simulink model "AGC"  (R2022a)
settings: Solver=FixedStepAuto  StartTime=0.0  StopTime=8000/Fs  RelTol=1e-3
undefined symbols (not defined in the file): a, alpha, Fixeda, FixedR, Fs, magnitude, R, TimeAxis
libraries: sim_stud_lib_r2022a x13, dspswit3 x2
settings Model: Creator=RolePyps  LastModifiedBy=RolePups
settings DebuggingCC: ParameterPrecisionLossMsg=none

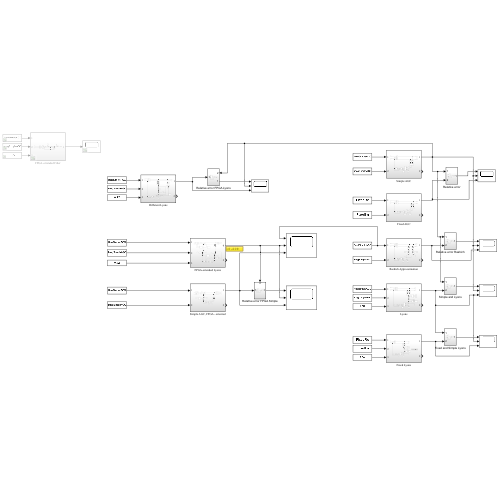
[thumbnail: Simulink's stored preview of the top-level diagram]
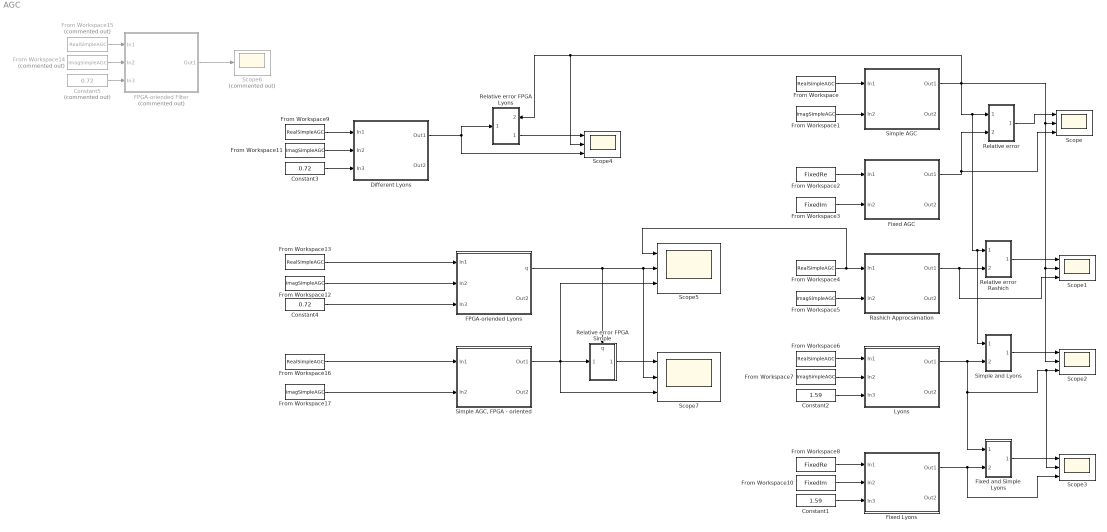
== system AGC ==
  Constant1 : Constant  Value=1.59  OutDataTypeStr=fixdt(0,13,11)  SampleTime=-1
  Constant2 : Constant  Value=1.59  SampleTime=1/Fs
  Constant3 : Constant  Value=0.72  SampleTime=1/Fs
  Constant4 : Constant  Value=0.72  SampleTime=TimeAxis(2)
  Constant5 : Constant  Commented=on  Value=0.72  SampleTime=1/Fs
  Different Lyons : Subsystem
  FPGA-oriended Filter : Subsystem  Commented=on
  FPGA-oriended Lyons : Subsystem
  Fixed AGC : Subsystem
  Fixed Lyons : Subsystem
  Fixed and Simple Lyons : Subsystem
  From Workspace{,4,6,9} (4 alike) : FromWorkspace  VariableName=RealSimpleAGC  OutDataTypeStr=double  SampleTime=1/Fs  Interpolate=off  OutputAfterFinalValue=Setting to zero
  From Workspace{1,5,7,11} (4 alike) : FromWorkspace  VariableName=ImagSimpleAGC  SampleTime=1/Fs  Interpolate=off  OutputAfterFinalValue=Setting to zero
  From Workspace10 : FromWorkspace  VariableName=FixedIm  OutDataTypeStr=fixdt(1,16,14)  SampleTime=1/Fs  Interpolate=off  OutputAfterFinalValue=Setting to zero
  From Workspace12 : FromWorkspace  VariableName=ImagSimpleAGC  SampleTime=TimeAxis(2)  Interpolate=off  OutputAfterFinalValue=Setting to zero
  From Workspace13 : FromWorkspace  VariableName=RealSimpleAGC  SampleTime=TimeAxis(2)  Interpolate=off  OutputAfterFinalValue=Setting to zero
  From Workspace14 : FromWorkspace  Commented=on  VariableName=ImagSimpleAGC  SampleTime=1/Fs  Interpolate=off  OutputAfterFinalValue=Setting to zero
  From Workspace15 : FromWorkspace  Commented=on  VariableName=RealSimpleAGC  OutDataTypeStr=double  SampleTime=1/Fs  Interpolate=off  OutputAfterFinalValue=Setting to zero
  From Workspace16 : FromWorkspace  VariableName=RealSimpleAGC  OutDataTypeStr=double  SampleTime=40/Fs  Interpolate=off  OutputAfterFinalValue=Setting to zero
  From Workspace17 : FromWorkspace  VariableName=ImagSimpleAGC  SampleTime=40/Fs  Interpolate=off  OutputAfterFinalValue=Setting to zero
  From Workspace2 : FromWorkspace  VariableName=FixedRe  OutDataTypeStr=fixdt(1,16,14)  SampleTime=1/Fs  Interpolate=off  OutputAfterFinalValue=Setting to zero
  From Workspace3 : FromWorkspace  VariableName=FixedIm  OutDataTypeStr=fixdt(1,16,14)  SampleTime=1/Fs  Interpolate=off  OutputAfterFinalValue=Setting to zero
  From Workspace8 : FromWorkspace  VariableName=FixedRe  OutDataTypeStr=fixdt(1,16,14)  SampleTime=1/Fs  Interpolate=off  OutputAfterFinalValue=Setting to zero
  Lyons : Subsystem
  Rashich Approcsimation : Subsystem
  Relative error : Subsystem
  Relative error FPGA Lyons : Subsystem
      settings: PortSchema="{\"entries\":[{\"content\":{\"sides\":[{\"content\":{\"connectorIds\":[\"In1\"]},\"type\":\"ConnectorPlacement.EquallySpacedRectSide\",\"uuid\":\"ab41bc29-8a88-48da-842a-7ea4b5d94515\"},{\"content\":{\"connectorIds\":[\"In2\",\"Out1\"],\"side\":\"RIGHT\"},\"type\":\"ConnectorPlacement.EquallySpacedRectSide\",\"uuid\":\"822f6f2f-923d-401a-b739-761bcd6fc88d\"},{\"content\":{\"connectorIds\":[],\"side\":\"TOP\"},\"type\":\"ConnectorPlacement.EquallySpacedRectSide\",\"uuid\":\"c3246772-222e-4e0d-9f9e-d4db37fa2bf2\"}]},\"type\":\"ConnectorPlacement.EquallySpacedConnector\",\"uuid\":\"7042a765-ada9-4885-ac85-35a265789643\"}],\"packageUris\":[\"http://schema.mathworks.com/mf0/Connector/R2020b\"],\"version\":\"1.0\"}"
  Relative error FPGA Simple : Subsystem
      settings: PortSchema="{\"entries\":[{\"content\":{\"sides\":[{\"content\":{\"connectorIds\":[\"In1\"]},\"type\":\"ConnectorPlacement.EquallySpacedRectSide\",\"uuid\":\"ab41bc29-8a88-48da-842a-7ea4b5d94515\"},{\"content\":{\"connectorIds\":[\"Out1\"],\"side\":\"RIGHT\"},\"type\":\"ConnectorPlacement.EquallySpacedRectSide\",\"uuid\":\"822f6f2f-923d-401a-b739-761bcd6fc88d\"},{\"content\":{\"connectorIds\":[\"In2\"],\"side\":\"TOP\"},\"type\":\"ConnectorPlacement.EquallySpacedRectSide\",\"uuid\":\"c3246772-222e-4e0d-9f9e-d4db37fa2bf2\"}]},\"type\":\"ConnectorPlacement.EquallySpacedConnector\",\"uuid\":\"7042a765-ada9-4885-ac85-35a265789643\"}],\"packageUris\":[\"http://schema.mathworks.com/mf0/Connector/R2020b\"],\"version\":\"1.0\"}"
  Relative error Rashich : Subsystem
  Scope{,1..5,7} (7 alike) : Scope  NumInputPorts=3
  Scope6 : Scope  Commented=on
  Simple AGC : Subsystem
  "Simple AGC, FPGA - oriented" : Subsystem
  Simple and Lyons : Subsystem
  wires:
  From Workspace/1 -> Simple AGC/1(In1)
  From Workspace1/1 -> Simple AGC/2(In2)
  Relative error/1(Out1) -> Scope/1
  From Workspace3/1 -> Fixed AGC/2(In2)
  From Workspace2/1 -> Fixed AGC/1(In1)
  Fixed AGC/1(Out1) -> Scope/3, Relative error/2(In3)
  From Workspace4/1 -> Scope5/1, Rashich Approcsimation/1(In1)
  From Workspace5/1 -> Rashich Approcsimation/2(In2)
  Rashich Approcsimation/1(Out1) -> Scope1/3, Relative error Rashich/2(In3)
  From Workspace6/1 -> Lyons/1(In1)
  From Workspace7/1 -> Lyons/2(In2)
  Lyons/1(Out1) -> Simple and Lyons/2(In3), Fixed and Simple Lyons/1(In1), Scope3/2, Scope2/3
  Simple and Lyons/1(Out1) -> Scope2/1
  Constant2/1 -> Lyons/3(In3)
  From Workspace8/1 -> Fixed Lyons/1(In1)
  Fixed Lyons/1(Out1) -> Fixed and Simple Lyons/2(In3), Scope3/3
  Constant1/1 -> Fixed Lyons/3(In3)
  From Workspace10/1 -> Fixed Lyons/2(In2)
  Fixed and Simple Lyons/1(Out1) -> Scope3/1
  Relative error Rashich/1(Out1) -> Scope1/1
  From Workspace11/1 -> Different Lyons/2(In2)
  Constant3/1 -> Different Lyons/3(In3)
  From Workspace9/1 -> Different Lyons/1(In1)
  Different Lyons/1(Out1) -> Scope4/3, Relative error FPGA Lyons/1(In3)
  Relative error FPGA Lyons/1(Out1) -> Scope4/1
  Constant4/1 -> FPGA-oriended Lyons/3(In3)
  From Workspace12/1 -> FPGA-oriended Lyons/2(In2)
  From Workspace15/1 -> FPGA-oriended Filter/1(In1)
  From Workspace14/1 -> FPGA-oriended Filter/2(In2)
  Constant5/1 -> FPGA-oriended Filter/3(In3)
  FPGA-oriended Filter/1(Out1) -> Scope6/1
  Simple AGC/1(Out1) -> Scope4/2, Relative error FPGA Lyons/2(In1), Scope2/2, Scope1/2, Scope/2, Simple and Lyons/1(In1), Relative error Rashich/1(In1), Relative error/1(In1)
  From Workspace13/1 -> FPGA-oriended Lyons/1(In1)
  FPGA-oriended Lyons/1(q) -> Relative error FPGA Simple/2(q), Scope7/2, Scope5/2
  From Workspace17/1 -> "Simple AGC, FPGA - oriented"/2(In2)
  From Workspace16/1 -> "Simple AGC, FPGA - oriented"/1(In1)
  "Simple AGC, FPGA - oriented"/1(Out1) -> Scope7/3, Relative error FPGA Simple/1(In3), Scope5/3
  Relative error FPGA Simple/1(Out1) -> Scope7/1

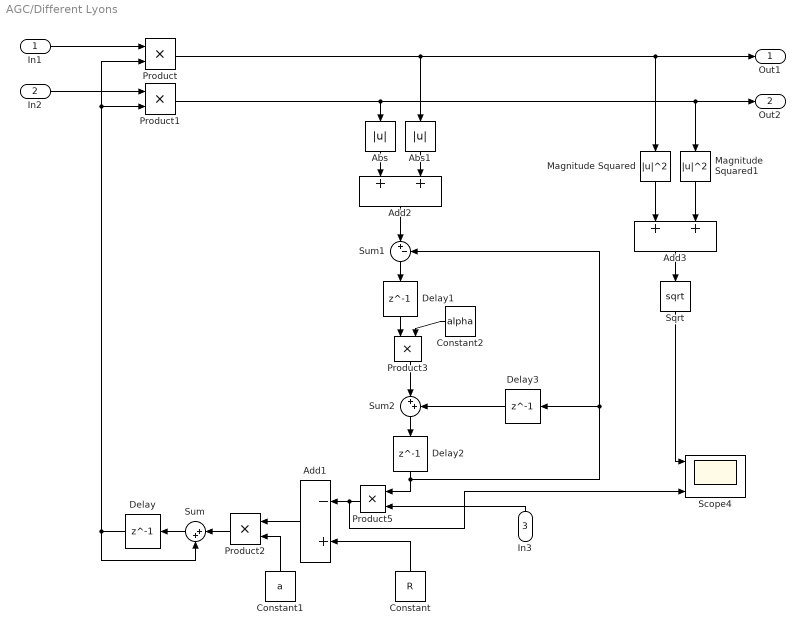
== system AGC/Different Lyons ==
  In1 : Inport
  In2 : Inport  Port=2
  In3 : Inport  Port=3  SampleTime=1/Fs
  Abs : Abs  SaturateOnIntegerOverflow=off
  Abs1 : Abs  SaturateOnIntegerOverflow=off
  Add1 : Sum  Inputs=-+  AccumDataTypeStr=double
  Add2 : Sum  AccumDataTypeStr=double
  Add3 : Sum  AccumDataTypeStr=double
  Constant : Constant  Value=R
  Constant1 : Constant  Value=a
  Constant2 : Constant  Value=alpha
  Delay{,1..3} (4 alike) : Delay  DelayLength=1  InitialCondition=0
  Magnitude Squared : Math  Operator=magnitude^2
  Magnitude Squared1 : Math  Operator=magnitude^2
  Product{,1..3,5} (5 alike) : Product  OutDataTypeStr=double
  Scope4 : Scope  NumInputPorts=3
  Sqrt : Sqrt
  Sum : Sum  Inputs=|++  AccumDataTypeStr=double
  Sum1 : Sum  Inputs=|+-  AccumDataTypeStr=double
  Sum2 : Sum  Inputs=|++  AccumDataTypeStr=double
  Out1 : Outport
  Out2 : Outport  Port=2
  wires:
  Delay/1 -> Sum/2, Product1/2, Product/2
  Product/1 -> Magnitude Squared/1, Out1/1, Abs1/1
  Add1/1 -> Product2/1
  Product1/1 -> Abs/1, Magnitude Squared1/1, Out2/1
  Constant/1 -> Add1/2
  In1/1 -> Product/1
  In2/1 -> Product1/1
  Sum/1 -> Delay/1
  Product2/1 -> Sum/1
  Constant1/1 -> Product2/2
  Abs1/1 -> Add2/2
  Abs/1 -> Add2/1
  In3/1 -> Product5/2
  Sum1/1 -> Delay1/1
  Product5/1 -> Scope4/3, Add1/1
  Add2/1 -> Sum1/1
  Delay1/1 -> Product3/1
  Constant2/1 -> Product3/2
  Product3/1 -> Sum2/1
  Sum2/1 -> Delay2/1
  Delay2/1 -> Delay3/1, Sum1/2, Product5/1
  Delay3/1 -> Sum2/2
  Magnitude Squared1/1 -> Add3/2
  Magnitude Squared/1 -> Add3/1
  Add3/1 -> Sqrt/1
  Sqrt/1 -> Scope4/1

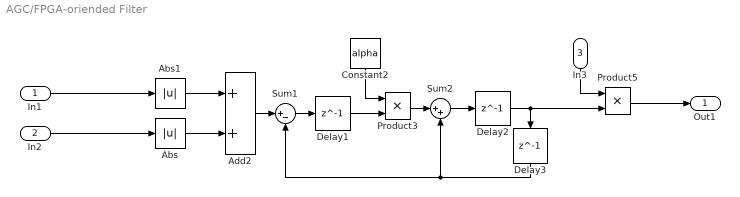
== system AGC/FPGA-oriended Filter ==
  In1 : Inport
  In2 : Inport  Port=2
  In3 : Inport  Port=3  SampleTime=1/Fs
  Abs : Abs  SaturateOnIntegerOverflow=off
  Abs1 : Abs  SaturateOnIntegerOverflow=off
  Add2 : Sum  AccumDataTypeStr=double
  Constant2 : Constant  Value=alpha
  Delay1 : Delay  DelayLength=1  InitialCondition=0
  Delay2 : Delay  DelayLength=1  InitialCondition=0
  Delay3 : Delay  DelayLength=1  InitialCondition=0
  Product3 : Product  OutDataTypeStr=double
  Product5 : Product  OutDataTypeStr=double
  Sum1 : Sum  Inputs=|+-  AccumDataTypeStr=double
  Sum2 : Sum  Inputs=|++  AccumDataTypeStr=double
  Out1 : Outport
  wires:
  Sum1/1 -> Delay1/1
  Add2/1 -> Sum1/1
  Product3/1 -> Sum2/1
  Sum2/1 -> Delay2/1
  Delay2/1 -> Product5/2, Delay3/1
  Delay3/1 -> Sum1/2, Sum2/2
  In3/1 -> Product5/1
  In1/1 -> Abs1/1
  In2/1 -> Abs/1
  Abs1/1 -> Add2/1
  Abs/1 -> Add2/2
  Delay1/1 -> Product3/2
  Constant2/1 -> Product3/1
  Product5/1 -> Out1/1

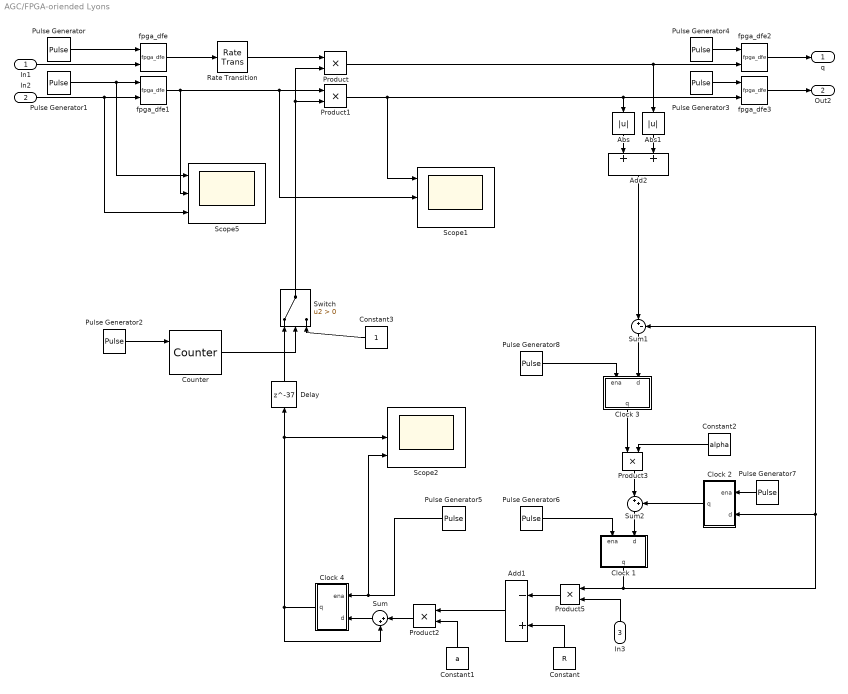
== system AGC/FPGA-oriended Lyons ==
  In1 : Inport
  In2 : Inport  Port=2
  In3 : Inport  Port=3  SampleTime=1/Fs
  Abs : Abs  SaturateOnIntegerOverflow=off
  Abs1 : Abs  SaturateOnIntegerOverflow=off
  Add1 : Sum  Inputs=-+  AccumDataTypeStr=double
  Add2 : Sum  AccumDataTypeStr=double
  Clock 1 : Subsystem
  Clock 2 : Subsystem
  Clock 3 : Subsystem
  Clock 4 : Subsystem
  Constant : Constant  Value=R
  Constant1 : Constant  Value=a
  Constant2 : Constant  Value=alpha
  Constant3 : Constant
  Counter : dspswit3/Counter  Direction=Up  CountEvent=Rising edge  CounterSize=User defined  MaxCount=1  InitialCount=0  Output=Count  HitValue=32  ResetInput=on  SamplesPerFrame=1  Ts=1  CntDtype=double  HitDtype=Logical
  Delay : Delay  DelayLength=37  InitialCondition=0  SampleTime=1/Fs
  Product{,1..3,5} (5 alike) : Product  OutDataTypeStr=double
  Pulse Generator : DiscretePulseGenerator  PulseType=Time based  Period=TimeAxis(2)  PulseWidth=50
  Pulse Generator1 : DiscretePulseGenerator  PulseType=Time based  Period=40/Fs  PulseWidth=50
  Pulse Generator2 : DiscretePulseGenerator  PulseType=Time based  Period=100  PulseWidth=50  PhaseDelay=80/Fs
  Pulse Generator3 : DiscretePulseGenerator  PulseType=Time based  Period=40/Fs  PulseWidth=50
  Pulse Generator4 : DiscretePulseGenerator  PulseType=Time based  Period=40/Fs  PulseWidth=50
  Pulse Generator5 : DiscretePulseGenerator  PulseType=Time based  Period=40/Fs  PulseWidth=2.5  PhaseDelay=42/Fs  VectorParams1D=off
  Pulse Generator6 : DiscretePulseGenerator  PulseType=Time based  Period=40/Fs  PulseWidth=2.5  PhaseDelay=1/Fs  VectorParams1D=off
  Pulse Generator7 : DiscretePulseGenerator  PulseType=Time based  Period=40/Fs  PulseWidth=2.5  PhaseDelay=2/Fs  VectorParams1D=off
  Pulse Generator8 : DiscretePulseGenerator  PulseType=Time based  Period=40/Fs  PulseWidth=2.5  VectorParams1D=off
  Rate Transition : RateTransition  OutPortSampleTime=TimeAxis(2)
  Scope1 : Scope  NumInputPorts=3
  Scope2 : Scope  NumInputPorts=3
  Scope5 : Scope  NumInputPorts=3
  Sum : Sum  Inputs=|++  AccumDataTypeStr=double
  Sum1 : Sum  Inputs=|+-  AccumDataTypeStr=double
  Sum2 : Sum  Inputs=|++  AccumDataTypeStr=double
  Switch : Switch  Criteria=u2 > Threshold  SaturateOnIntegerOverflow=off  InputSameDT=off
  fpga_dfe{,1..3} (4 alike) : sim_stud_lib_r2022a/fpga_dfe  SystemSampleTime=-1  VariantActivationTime=update diagram  Latency=0  AutoFrameSizeCalculation=off
  q : Outport
  Out2 : Outport  Port=2
  wires:
  Clock 4/1(q) -> Sum/2, Delay/1, Scope2/2
  Product/1 -> Abs1/1, fpga_dfe2/2
  Product1/1 -> Scope1/1, fpga_dfe3/2, Abs/1
  Constant/1 -> Add1/2
  Sum/1 -> Clock 4/2(d)
  Product2/1 -> Sum/1
  Constant1/1 -> Product2/2
  Abs1/1 -> Add2/2
  Abs/1 -> Add2/1
  In3/1 -> Product5/2
  Sum1/1 -> Clock 3/2(d)
  Product5/1 -> Add1/1
  Constant2/1 -> Product3/2
  Product3/1 -> Sum2/1
  Clock 2/1(q) -> Sum2/2
  Pulse Generator/1 -> fpga_dfe/1
  In1/1 -> fpga_dfe/2
  In2/1 -> Scope5/3, fpga_dfe1/2
  fpga_dfe/1 -> Rate Transition/1
  Rate Transition/1 -> Product/1
  fpga_dfe1/1 -> Scope1/2, Product1/1, Scope5/2
  Pulse Generator1/1 -> Scope5/1, fpga_dfe1/1
  Add1/1 -> Product2/1
  Constant3/1 -> Switch/3
  Switch/1 -> Product/2, Product1/2
  Counter/1 -> Switch/2
  Pulse Generator2/1 -> Counter/1
  Sum2/1 -> Clock 1/2(d)
  Clock 1/1(q) -> Product5/1, Sum1/2, Clock 2/2(d)
  Pulse Generator6/1 -> Clock 1/1(ena)
  Pulse Generator7/1 -> Clock 2/1(ena)
  Clock 3/1(q) -> Product3/1
  Pulse Generator8/1 -> Clock 3/1(ena)
  Add2/1 -> Sum1/1
  Pulse Generator5/1 -> Scope2/3, Clock 4/1(ena)
  Delay/1 -> Switch/1
  Pulse Generator4/1 -> fpga_dfe2/1
  fpga_dfe2/1 -> q/1
  Pulse Generator3/1 -> fpga_dfe3/1
  fpga_dfe3/1 -> Out2/1

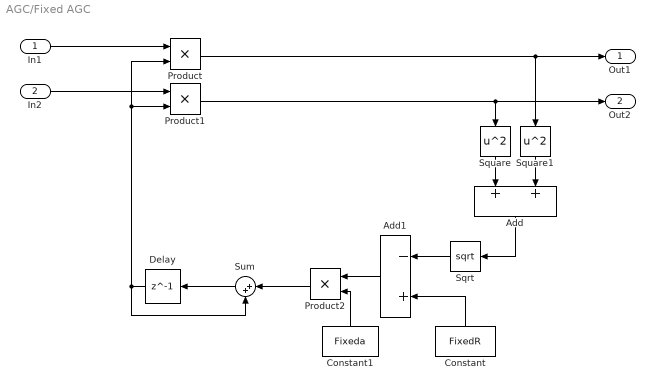
== system AGC/Fixed AGC ==
  In1 : Inport
  In2 : Inport  Port=2
  Add : Sum  AccumDataTypeStr=fixdt(1,34,22)  OutDataTypeStr=double
  Add1 : Sum  Inputs=-+  AccumDataTypeStr=fixdt(1,19,11)
  Constant : Constant  Value=FixedR
  Constant1 : Constant  Value=Fixeda
  Delay : Delay  DelayLength=1  InitialCondition=0  SampleTime=1/Fs
  Product : Product  OutDataTypeStr=fixdt(1,16,11)
  Product1 : Product  OutDataTypeStr=fixdt(1,16,11)
  Product2 : Product  OutDataTypeStr=fixdt(1,25,16)
  Sqrt : Sqrt  OutDataTypeStr=fixdt(1,18,11)
  Square : Math  Operator=square  OutDataTypeStr=fixdt(1,33,22)
  Square1 : Math  Operator=square  OutDataTypeStr=fixdt(1,33,22)
  Sum : Sum  Inputs=|++  OutDataTypeStr=fixdt(1,25,16)
  Out1 : Outport
  Out2 : Outport  Port=2
  wires:
  Square/1 -> Add/1
  Sqrt/1 -> Add1/1
  Delay/1 -> Sum/2, Product/2, Product1/2
  Product/1 -> Out1/1, Square1/1
  Add1/1 -> Product2/1
  Product1/1 -> Out2/1, Square/1
  Constant/1 -> Add1/2
  In1/1 -> Product/1
  In2/1 -> Product1/1
  Sum/1 -> Delay/1
  Product2/1 -> Sum/1
  Square1/1 -> Add/2
  Add/1 -> Sqrt/1
  Constant1/1 -> Product2/2

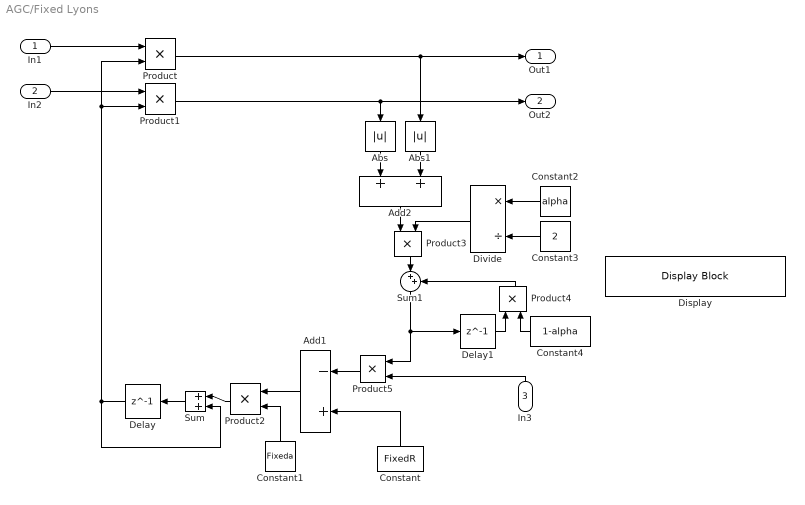
== system AGC/Fixed Lyons ==
  In1 : Inport
  In2 : Inport  Port=2
  In3 : Inport  Port=3  OutDataTypeStr=fixdt(0,13,11)  SampleTime=1/Fs
  Abs : Abs  OutDataTypeStr=fixdt(0,16,11)  SaturateOnIntegerOverflow=off
  Abs1 : Abs  OutDataTypeStr=fixdt(0,16,11)  SaturateOnIntegerOverflow=off
  Add1 : Sum  Inputs=-+  AccumDataTypeStr=double  OutDataTypeStr=fixdt(1,25,16)
  Add2 : Sum  AccumDataTypeStr=fixdt(1,17,11)
  Constant : Constant  Value=FixedR
  Constant1 : Constant  Value=Fixeda  OutDataTypeStr=fixdt(1,13,12)  SampleTime=1/Fs
  Constant2 : Constant  Value=alpha  OutDataTypeStr=fixdt(0,6,6)
  Constant3 : Constant  Value=2  OutDataTypeStr=fixdt(0,2,0)  SampleTime=1/Fs  LockScale=on
  Constant4 : Constant  Value=1-alpha  OutDataTypeStr=fixdt(0,6,6)
  Delay : Delay  DelayLength=1  InitialCondition=0
  Delay1 : Delay  DelayLength=1  InitialCondition=0
  Display : DisplayBlock  LabelPosition=Hide  Transparency=1  Layout=Fill available space
  Divide : Product  Inputs=*/  OutDataTypeStr=fixdt(0,6,6)  LockScale=on
  Product : Product  OutDataTypeStr=fixdt(1,16,11)
  Product1 : Product  OutDataTypeStr=fixdt(1,16,11)
  Product2 : Product  OutDataTypeStr=fixdt(1,25,16)
  Product3 : Product  OutDataTypeStr=fixdt(1,17,11)
  Product4 : Product  OutDataTypeStr=fixdt(1,25,16)
  Product5 : Product  OutDataTypeStr=fixdt(1,25,16)
  Sum : Sum  Inputs=|++  AccumDataTypeStr=fixdt(1,25,16)  OutDataTypeStr=fixdt(1,25,16)
  Sum1 : Sum  Inputs=|++  AccumDataTypeStr=fixdt(1,25,16)  OutDataTypeStr=fixdt(1,25,16)
  Out1 : Outport
  Out2 : Outport  Port=2
  wires:
  Delay/1 -> Sum/2, Product1/2, Product/2
  Product/1 -> Out1/1, Abs1/1
  Add1/1 -> Product2/1
  Product1/1 -> Abs/1, Out2/1
  Constant/1 -> Add1/2
  In1/1 -> Product/1
  In2/1 -> Product1/1
  Sum/1 -> Delay/1
  Product2/1 -> Sum/1
  Constant1/1 -> Product2/2
  Abs1/1 -> Add2/2
  Abs/1 -> Add2/1
  Add2/1 -> Product3/1
  Constant2/1 -> Divide/1
  Constant3/1 -> Divide/2
  Divide/1 -> Product3/2
  Product3/1 -> Sum1/1
  In3/1 -> Product5/2
  Sum1/1 -> Delay1/1, Product5/1
  Product5/1 -> Add1/1
  Delay1/1 -> Product4/1
  Constant4/1 -> Product4/2
  Product4/1 -> Sum1/2

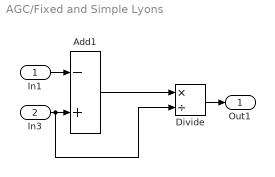
== system AGC/Fixed and Simple Lyons ==
  In1 : Inport
  In3 : Inport  Port=2
  Add1 : Sum  Inputs=-+  AccumDataTypeStr=double
  Divide : Product  Inputs=*/
  Out1 : Outport
  wires:
  Add1/1 -> Divide/1
  In3/1 -> Divide/2, Add1/2
  Divide/1 -> Out1/1
  In1/1 -> Add1/1

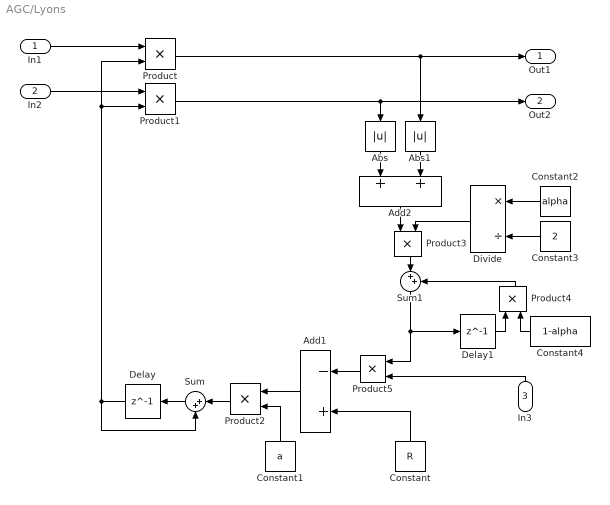
== system AGC/Lyons ==
  In1 : Inport
  In2 : Inport  Port=2
  In3 : Inport  Port=3  SampleTime=1/Fs
  Abs : Abs  SaturateOnIntegerOverflow=off
  Abs1 : Abs  SaturateOnIntegerOverflow=off
  Add1 : Sum  Inputs=-+  AccumDataTypeStr=double
  Add2 : Sum  AccumDataTypeStr=double
  Constant : Constant  Value=R
  Constant1 : Constant  Value=a
  Constant2 : Constant  Value=alpha
  Constant3 : Constant  Value=2
  Constant4 : Constant  Value=1-alpha
  Delay : Delay  DelayLength=1  InitialCondition=0
  Delay1 : Delay  DelayLength=1  InitialCondition=0
  Divide : Product  Inputs=*/
  Product{,1..5} (6 alike) : Product  OutDataTypeStr=double
  Sum : Sum  Inputs=|++  AccumDataTypeStr=double
  Sum1 : Sum  Inputs=|++  AccumDataTypeStr=double
  Out1 : Outport
  Out2 : Outport  Port=2
  wires:
  Delay/1 -> Sum/2, Product1/2, Product/2
  Product/1 -> Out1/1, Abs1/1
  Add1/1 -> Product2/1
  Product1/1 -> Abs/1, Out2/1
  Constant/1 -> Add1/2
  In1/1 -> Product/1
  In2/1 -> Product1/1
  Sum/1 -> Delay/1
  Product2/1 -> Sum/1
  Constant1/1 -> Product2/2
  Abs1/1 -> Add2/2
  Abs/1 -> Add2/1
  Add2/1 -> Product3/1
  Constant2/1 -> Divide/1
  Constant3/1 -> Divide/2
  Divide/1 -> Product3/2
  Product3/1 -> Sum1/1
  In3/1 -> Product5/2
  Sum1/1 -> Delay1/1, Product5/1
  Product5/1 -> Add1/1
  Delay1/1 -> Product4/1
  Constant4/1 -> Product4/2
  Product4/1 -> Sum1/2

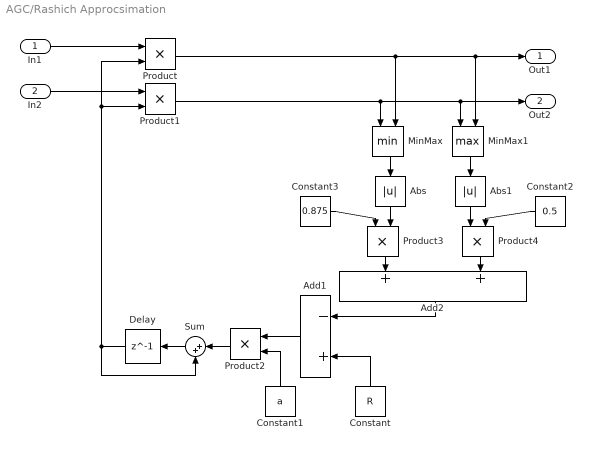
== system AGC/Rashich Approcsimation ==
  In1 : Inport
  In2 : Inport  Port=2
  Abs : Abs  SaturateOnIntegerOverflow=off
  Abs1 : Abs  SaturateOnIntegerOverflow=off
  Add1 : Sum  Inputs=-+  AccumDataTypeStr=double
  Add2 : Sum  AccumDataTypeStr=double
  Constant : Constant  Value=R
  Constant1 : Constant  Value=a
  Constant2 : Constant  Value=0.5
  Constant3 : Constant  Value=0.875
  Delay : Delay  DelayLength=1  InitialCondition=0
  MinMax : MinMax  Inputs=2
  MinMax1 : MinMax  Function=max  Inputs=2
  Product{,1..4} (5 alike) : Product  OutDataTypeStr=double
  Sum : Sum  Inputs=|++  AccumDataTypeStr=double
  Out1 : Outport
  Out2 : Outport  Port=2
  wires:
  Delay/1 -> Sum/2, Product1/2, Product/2
  Product/1 -> MinMax/2, MinMax1/2, Out1/1
  Add1/1 -> Product2/1
  Product1/1 -> MinMax/1, MinMax1/1, Out2/1
  Constant/1 -> Add1/2
  In1/1 -> Product/1
  In2/1 -> Product1/1
  Sum/1 -> Delay/1
  Product2/1 -> Sum/1
  Constant1/1 -> Product2/2
  MinMax/1 -> Abs/1
  MinMax1/1 -> Abs1/1
  Abs/1 -> Product3/2
  Constant3/1 -> Product3/1
  Abs1/1 -> Product4/1
  Constant2/1 -> Product4/2
  Product3/1 -> Add2/1
  Product4/1 -> Add2/2
  Add2/1 -> Add1/1

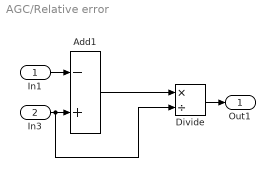
== system AGC/Relative error ==
  In1 : Inport
  In3 : Inport  Port=2
  Add1 : Sum  Inputs=-+  AccumDataTypeStr=double
  Divide : Product  Inputs=*/
  Out1 : Outport
  wires:
  Add1/1 -> Divide/1
  In3/1 -> Divide/2, Add1/2
  Divide/1 -> Out1/1
  In1/1 -> Add1/1

== system AGC/Relative error FPGA Lyons ==
  In3 : Inport
  In1 : Inport  Port=2
  Add1 : Sum  Inputs=-+  AccumDataTypeStr=double
  Divide : Product  Inputs=*/
  Out1 : Outport
  wires:
  Add1/1 -> Divide/1
  In3/1 -> Divide/2, Add1/2
  Divide/1 -> Out1/1
  In1/1 -> Add1/1

== system AGC/Relative error FPGA Simple ==
  In3 : Inport
  q : Inport  Port=2
  Add1 : Sum  Inputs=-+  AccumDataTypeStr=double
  Divide : Product  Inputs=*/
  Out1 : Outport
  wires:
  Add1/1 -> Divide/1
  In3/1 -> Divide/2, Add1/2
  Divide/1 -> Out1/1
  q/1 -> Add1/1

== system AGC/Relative error Rashich ==
  In1 : Inport
  In3 : Inport  Port=2
  Add1 : Sum  Inputs=-+  AccumDataTypeStr=double
  Divide : Product  Inputs=*/
  Out1 : Outport
  wires:
  Add1/1 -> Divide/1
  In3/1 -> Divide/2, Add1/2
  Divide/1 -> Out1/1
  In1/1 -> Add1/1

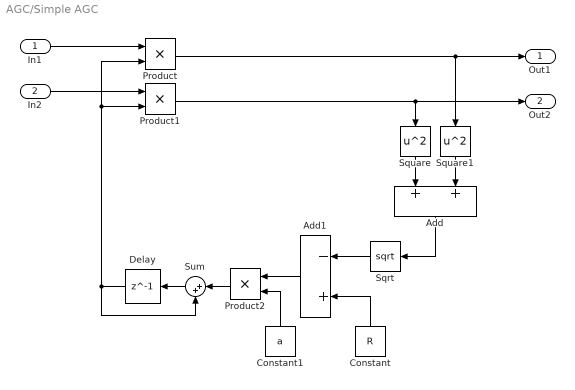
== system AGC/Simple AGC ==
  In1 : Inport
  In2 : Inport  Port=2
  Add : Sum  OutDataTypeStr=double
  Add1 : Sum  Inputs=-+  AccumDataTypeStr=double
  Constant : Constant  Value=R
  Constant1 : Constant  Value=a
  Delay : Delay  DelayLength=1  InitialCondition=0
  Product : Product  OutDataTypeStr=double
  Product1 : Product  OutDataTypeStr=double
  Product2 : Product  OutDataTypeStr=double
  Sqrt : Sqrt  OutDataTypeStr=double
  Square : Math  Operator=square  OutDataTypeStr=double
  Square1 : Math  Operator=square  OutDataTypeStr=double
  Sum : Sum  Inputs=|++  AccumDataTypeStr=double
  Out1 : Outport
  Out2 : Outport  Port=2
  wires:
  Square/1 -> Add/1
  Sqrt/1 -> Add1/1
  Delay/1 -> Sum/2, Product1/2, Product/2
  Product/1 -> Out1/1, Square1/1
  Add1/1 -> Product2/1
  Product1/1 -> Out2/1, Square/1
  Constant/1 -> Add1/2
  In1/1 -> Product/1
  In2/1 -> Product1/1
  Sum/1 -> Delay/1
  Product2/1 -> Sum/1
  Square1/1 -> Add/2
  Add/1 -> Sqrt/1
  Constant1/1 -> Product2/2

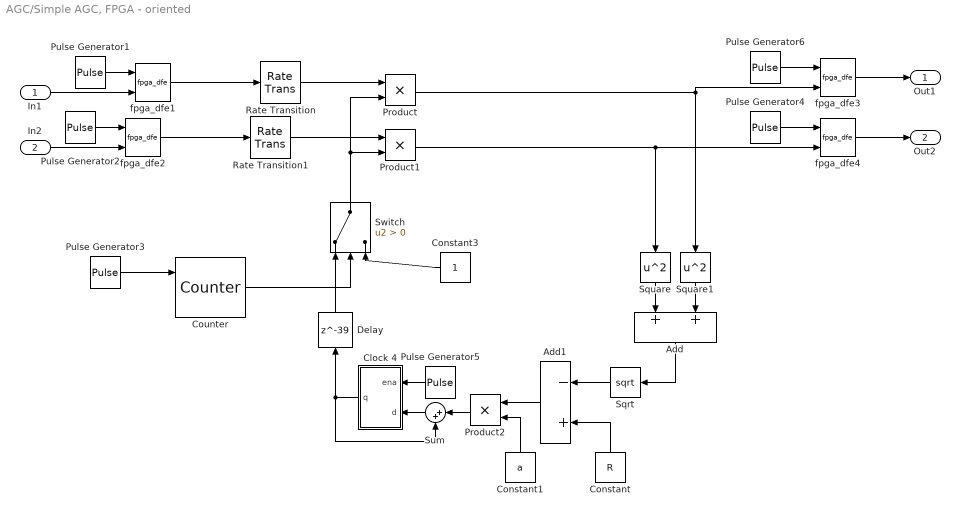
== system AGC/Simple AGC, FPGA - oriented ==
  In1 : Inport
  In2 : Inport  Port=2
  Add : Sum  OutDataTypeStr=double
  Add1 : Sum  Inputs=-+  AccumDataTypeStr=double
  Clock 4 : Subsystem
  Constant : Constant  Value=R
  Constant1 : Constant  Value=a
  Constant3 : Constant
  Counter : dspswit3/Counter  Direction=Up  CountEvent=Rising edge  CounterSize=User defined  MaxCount=1  InitialCount=0  Output=Count  HitValue=32  ResetInput=on  SamplesPerFrame=1  Ts=1  CntDtype=double  HitDtype=Logical
  Delay : Delay  DelayLength=39  InitialCondition=0  SampleTime=1/Fs
  Product : Product  OutDataTypeStr=double
  Product1 : Product  OutDataTypeStr=double
  Product2 : Product  OutDataTypeStr=double
  Pulse Generator{1..2,4,6} (4 alike) : DiscretePulseGenerator  PulseType=Time based  Period=40/Fs  PulseWidth=50
  Pulse Generator3 : DiscretePulseGenerator  PulseType=Time based  Period=100  PulseWidth=50  PhaseDelay=80/Fs
  Pulse Generator5 : DiscretePulseGenerator  PulseType=Time based  Period=40/Fs  PulseWidth=2.5  PhaseDelay=40/Fs  VectorParams1D=off
  Rate Transition : RateTransition  OutPortSampleTime=TimeAxis(2)
  Rate Transition1 : RateTransition  OutPortSampleTime=TimeAxis(2)
  Sqrt : Sqrt  OutDataTypeStr=double
  Square : Math  Operator=square  OutDataTypeStr=double
  Square1 : Math  Operator=square  OutDataTypeStr=double
  Sum : Sum  Inputs=|++  AccumDataTypeStr=double
  Switch : Switch  Criteria=u2 > Threshold  SaturateOnIntegerOverflow=off  InputSameDT=off
  fpga_dfe{1..4} (4 alike) : sim_stud_lib_r2022a/fpga_dfe  SystemSampleTime=-1  VariantActivationTime=update diagram  Latency=0  AutoFrameSizeCalculation=off
  Out1 : Outport
  Out2 : Outport  Port=2
  wires:
  Square/1 -> Add/1
  Sqrt/1 -> Add1/1
  Add1/1 -> Product2/1
  Constant/1 -> Add1/2
  Sum/1 -> Clock 4/2(d)
  Product2/1 -> Sum/1
  Square1/1 -> Add/2
  Add/1 -> Sqrt/1
  Constant1/1 -> Product2/2
  Pulse Generator1/1 -> fpga_dfe1/1
  In1/1 -> fpga_dfe1/2
  Pulse Generator2/1 -> fpga_dfe2/1
  In2/1 -> fpga_dfe2/2
  Pulse Generator5/1 -> Clock 4/1(ena)
  Pulse Generator3/1 -> Counter/1
  Counter/1 -> Switch/2
  Constant3/1 -> Switch/3
  Clock 4/1(q) -> Delay/1, Sum/2
  Switch/1 -> Product/2, Product1/2
  Delay/1 -> Switch/1
  fpga_dfe1/1 -> Rate Transition/1
  Rate Transition/1 -> Product/1
  Rate Transition1/1 -> Product1/1
  fpga_dfe2/1 -> Rate Transition1/1
  Product/1 -> Square1/1, fpga_dfe3/2
  Pulse Generator4/1 -> fpga_dfe4/1
  Product1/1 -> Square/1, fpga_dfe4/2
  fpga_dfe4/1 -> Out2/1
  Pulse Generator6/1 -> fpga_dfe3/1
  fpga_dfe3/1 -> Out1/1

== system AGC/Simple and Lyons ==
  In1 : Inport
  In3 : Inport  Port=2
  Add1 : Sum  Inputs=-+  AccumDataTypeStr=double
  Divide : Product  Inputs=*/
  Out1 : Outport
  wires:
  Add1/1 -> Divide/1
  In3/1 -> Divide/2, Add1/2
  Divide/1 -> Out1/1
  In1/1 -> Add1/1

== system AGC/FPGA-oriended Lyons/Clock 1 ==
  ena : Inport
  d : Inport  Port=2
  Delay16 : Delay  DelayLength=1  SampleTime=1/Fs
  Enabled Subsystem : sim_stud_lib_r2022a/fpga_dfe/Enabled Subsystem  SystemSampleTime=-1  VariantActivationTime=update diagram  Latency=0  AutoFrameSizeCalculation=off
  q : Outport  VectorParamsAs1DForOutWhenUnconnected=off
  wires:
  Delay16/1 -> q/1
  d/1 -> Enabled Subsystem/1
  Enabled Subsystem/1 -> Delay16/1
  ena/1 -> Enabled Subsystem/Enable

== system AGC/FPGA-oriended Lyons/Clock 2 ==
  ena : Inport
  d : Inport  Port=2
  Delay16 : Delay  DelayLength=1  SampleTime=1/Fs
  Enabled Subsystem : sim_stud_lib_r2022a/fpga_dfe/Enabled Subsystem  SystemSampleTime=-1  VariantActivationTime=update diagram  Latency=0  AutoFrameSizeCalculation=off
  q : Outport  VectorParamsAs1DForOutWhenUnconnected=off
  wires:
  Delay16/1 -> q/1
  d/1 -> Enabled Subsystem/1
  Enabled Subsystem/1 -> Delay16/1
  ena/1 -> Enabled Subsystem/Enable

== system AGC/FPGA-oriended Lyons/Clock 3 ==
  ena : Inport
  d : Inport  Port=2
  Delay16 : Delay  DelayLength=1  SampleTime=1/Fs
  Enabled Subsystem : sim_stud_lib_r2022a/fpga_dfe/Enabled Subsystem  SystemSampleTime=-1  VariantActivationTime=update diagram  Latency=0  AutoFrameSizeCalculation=off
  q : Outport  VectorParamsAs1DForOutWhenUnconnected=off
  wires:
  Delay16/1 -> q/1
  d/1 -> Enabled Subsystem/1
  Enabled Subsystem/1 -> Delay16/1
  ena/1 -> Enabled Subsystem/Enable

== system AGC/FPGA-oriended Lyons/Clock 4 ==
  ena : Inport
  d : Inport  Port=2
  Delay16 : Delay  DelayLength=1  SampleTime=1/Fs
  Enabled Subsystem : sim_stud_lib_r2022a/fpga_dfe/Enabled Subsystem  SystemSampleTime=-1  VariantActivationTime=update diagram  Latency=0  AutoFrameSizeCalculation=off
  q : Outport  VectorParamsAs1DForOutWhenUnconnected=off
  wires:
  Delay16/1 -> q/1
  d/1 -> Enabled Subsystem/1
  Enabled Subsystem/1 -> Delay16/1
  ena/1 -> Enabled Subsystem/Enable

== system AGC/Simple AGC, FPGA - oriented/Clock 4 ==
  ena : Inport
  d : Inport  Port=2
  Delay16 : Delay  DelayLength=1  SampleTime=1/Fs
  Enabled Subsystem : sim_stud_lib_r2022a/fpga_dfe/Enabled Subsystem  SystemSampleTime=-1  VariantActivationTime=update diagram  Latency=0  AutoFrameSizeCalculation=off
  q : Outport  VectorParamsAs1DForOutWhenUnconnected=off
  wires:
  Delay16/1 -> q/1
  d/1 -> Enabled Subsystem/1
  Enabled Subsystem/1 -> Delay16/1
  ena/1 -> Enabled Subsystem/Enable
